simulink library "fro"  (Simulink 8.1)
settings: Solver=ode1  StartTime=0.0  StopTime=Inf  FixedStep=0.001  RelTol=1e-3
PostLoadFcn:
  | , if any(exist('dsrtsu_mdlpostloadfcn', 'file') == [2, 3, 6]), try dsrtsu_mdlpostloadfcn('Execute', bdroot); catch fprintf('Error in PostLoadFcn (dsrtsu_mdlpostloadfcn) for model "%s":\n %s\n', bdroot, lasterr); end, end,
undefined symbols (not defined in the file or in its folder): KJUD_FCWReturnOpRelSpeedX_kph, KJUD_FCWReturnOpVehClearance_m
libraries: hcu_lib x1
settings Model: DSRTSU_INTERNAL_RTI_VER=450  DSRTSU_INTERNAL_RTI_TYPE=rti1401  RTICANMMDATA=struct('GeneralSetupData',struct('modelroot','D:\PROJECTS\HAITEC\TAIWAN_HAITEC_SVN\trunk\AdasDragon\software\sw_development\arch\app\jud','generalsettings',struct('filesettings',struct('destfolder',struct('Name','RTICANMM_FILES','Check',1),'buildfolder',struct('Name','.','Check',1),'AbsDestfolder',struct('Name','D:\PROJECTS\HAITEC\TAIWAN_HAITEC_SVN\trunk\AdasDragon\software\sw_development\arch\app\jud\RTICANMM_FILES'),'AbsBuildfolder',struct('Name','D:\PROJECTS\HAITEC\TAIWAN_HAITEC_SVN\trunk\AdasDragon\software\sw_development\arch\app\jud'))),'options',struct('addpaths',1,'rmpaths',1,'addtrcexclusion',logical(1),'cannavigator',struct('checkmonitoring',0),'show_usrtrc',0,'use_usrtrc',0),'advanced',struct('options',[1 1 1 1 1 1 1 1 1 1 1 1 1 1 1 1 1 1 1 1 1 1 1 1 1 1 1 1 1 1 1 1 1 1 1 1 1 1 1 1 1 1 1 1 1 1 1 1 1 1 1 1 1 1 1 1 1 1 1 1 1 1 1 1 1 1 1 1 1 1 1 1 1 1 1 1 1 1 1 1 1 1 1 1 1 1 1 1 1 1 1 1 1 1 1 1 1 1 1 1]),'MPSetup',{{}},'modelname','fro','block','fro'))  DSRTSU_INTERNAL_RTIFPGA=40  Creator=AT015411  LastModifiedBy=tescamilla

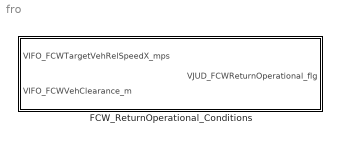
== system fro ==
  FCW_ReturnOperational_Conditions : Subsystem

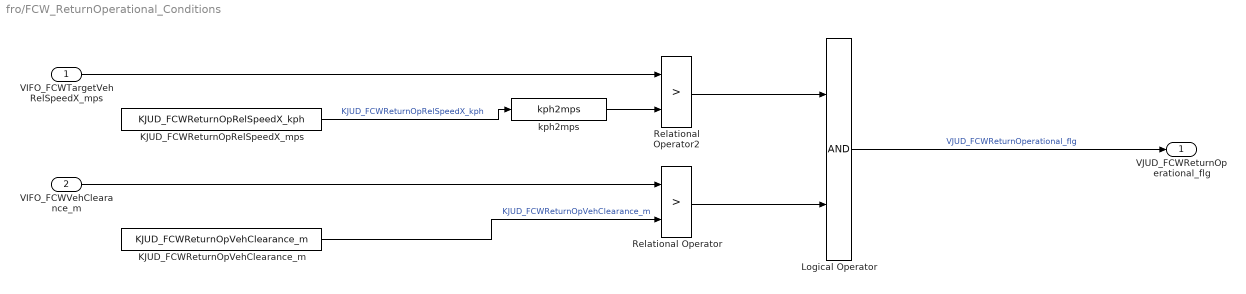
== system fro/FCW_ReturnOperational_Conditions ==
  VIFO_FCWTargetVehRelSpeedX_mps : Inport
  VIFO_FCWVehClearance_m : Inport  Port=2
  KJUD_FCWReturnOpRelSpeedX_mps : Constant  Value=KJUD_FCWReturnOpRelSpeedX_kph
  KJUD_FCWReturnOpVehClearance_m : Constant  Value=KJUD_FCWReturnOpVehClearance_m
  Logical Operator : Logic  AllPortsSameDT=off  OutDataTypeStr=boolean
  Relational Operator : RelationalOperator  Operator=>  OutDataTypeStr=boolean
  Relational Operator2 : RelationalOperator  Operator=>  OutDataTypeStr=boolean
  kph2mps : hcu_lib/kph2mps
  VJUD_FCWReturnOperational_flg : Outport
  wires:
  VIFO_FCWVehClearance_m/1 -> Relational Operator/1
  KJUD_FCWReturnOpVehClearance_m/1 -> Relational Operator/2  "KJUD_FCWReturnOpVehClearance_m"
  Logical Operator/1 -> VJUD_FCWReturnOperational_flg/1  "VJUD_FCWReturnOperational_flg"
  KJUD_FCWReturnOpRelSpeedX_mps/1 -> kph2mps/1  "KJUD_FCWReturnOpRelSpeedX_kph"
  Relational Operator/1 -> Logical Operator/2
  Relational Operator2/1 -> Logical Operator/1
  VIFO_FCWTargetVehRelSpeedX_mps/1 -> Relational Operator2/1
  kph2mps/1 -> Relational Operator2/2
